simulink model "sensor_system"  (R2021b)
settings: Solver=VariableStepAuto  StartTime=0.0  StopTime=10  RelTol=1e-3
libraries: slpidlib x1, simulink x1
settings Model: Creator=mluser  LastModifiedBy=mluser

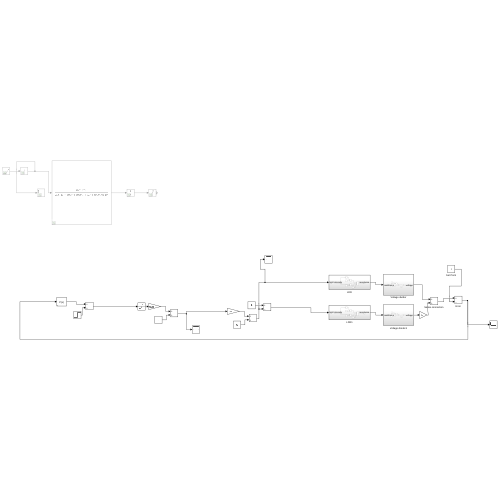
[thumbnail: Simulink's stored preview of the top-level diagram]
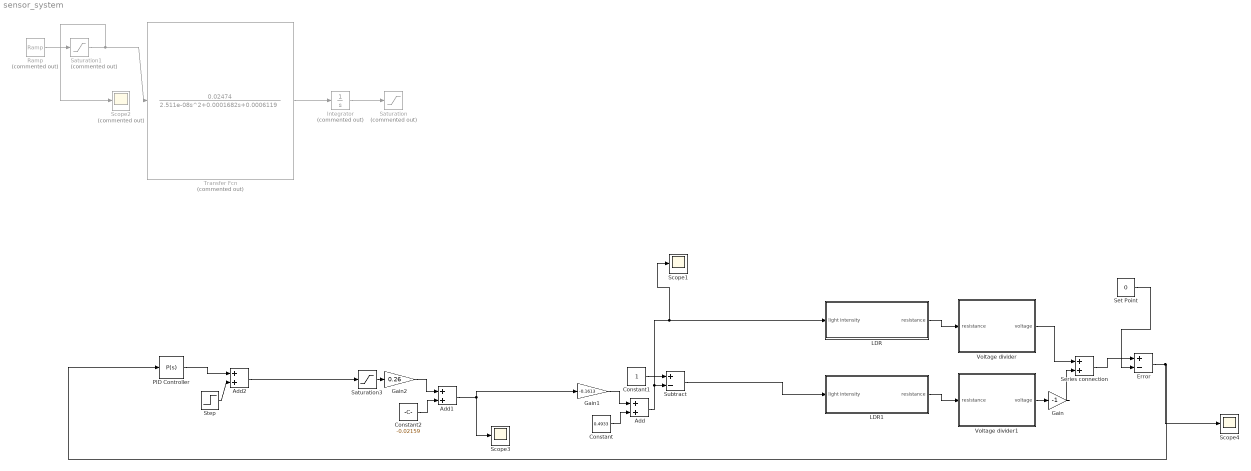
== system sensor_system ==
  Add : Sum
  Add1 : Sum
  Add2 : Sum
  Constant : Constant  Value=0.4933
  Constant1 : Constant
  Constant2 : Constant  Value=-0.02159
  Error : Sum  Inputs=+-
  Gain : Gain  Gain=-1
  Gain1 : Gain  Gain=-0.1613
  Gain2 : Gain  Gain=0.26
  Integrator : Integrator  Commented=on
  LDR : Subsystem
  LDR1 : Subsystem
  PID Controller : slpidlib/PID Controller  Controller=P  Form=Parallel  TimeDomain=Continuous-time  UseExternalTs=off  SampleTime=-1  IntegratorMethod=Forward Euler  FilterMethod=Forward Euler  ControllerParametersSource=internal  P=0.8  I=1  D=0.1  UseFilter=on  N=100  TunerSelectOption=Transfer Function Based (PID Tuner App)  InitialConditionSource=internal  InitialConditionForIntegrator=0  InitialConditionForFilter=0  DifferentiatorICPrevScaledInput=0  ExternalReset=none  TrackingMode=off  Kt=1  LimitOutput=off  SatLimitsSource=internal  UpperSaturationLimit=inf  LowerSaturationLimit=-inf  LinearizeAsGain=on  AntiWindupMode=none  Kb=1  POutMin=[]  POutMax=[]  IOutMin=[]  IOutMax=[]  DOutMin=[]  DOutMax=[]  NOutMin=[]  NOutMax=[]  SumOutMin=[]  SumOutMax=[]  SaturationOutMin=[]  SaturationOutMax=[]  PParamMin=[]  PParamMax=[]  IParamMin=[]  IParamMax=[]  DParamMin=[]  DParamMax=[]  NParamMin=[]  NParamMax=[]  KbParamMin=[]  KbParamMax=[]  KtParamMin=[]  KtParamMax=[]  KbOutMin=[]  KbOutMax=[]  KtOutMin=[]  KtOutMax=[]  IntegratorOutMin=[]  IntegratorOutMax=[]  FilterOutMin=[]  FilterOutMax=[]  SumI1OutMin=[]  SumI1OutMax=[]  SumI2OutMin=[]  SumI2OutMax=[]  SumI3OutMin=[]  SumI3OutMax=[]  SumI4OutMin=[]  SumI4OutMax=[]  SumDOutMin=[]  SumDOutMax=[]  DifferentiatorOutMin=[]  DifferentiatorOutMax=[]  FilterDiffOutCoefMin=[]  FilterDiffOutCoefMax=[]  ReciprocalOutMin=[]  ReciprocalOutMax=[]  SumDenOutMin=[]  SumDenOutMax=[]  SumNumOutMin=[]  SumNumOutMax=[]  DivideOutMin=[]  DivideOutMax=[]  UdiffTsProdOutMin=[]  UdiffTsProdOutMax=[]  NTsProdOutMin=[]  NTsProdOutMax=[]  UintegralTsProdOutMin=[]  UintegralTsProdOutMax=[]  UngainTsProdOutMin=[]  UngainTsProdOutMax=[]  IntegratorContinuousStateAttributes=''  IntegratorStateMustResolveToSignalObject=off  IntegratorRTWStateStorageClass=Auto  FilterContinuousStateAttributes=''  FilterStateMustResolveToSignalObject=off  FilterRTWStateStorageClass=Auto  ParallelPVariant=InternalParameters  IdealPVariant=Disabled  IVariant=Disabled  DVariant=Disabled  IntegratorVariant=Disabled  SatVariant=Disabled  AWVariant=Disabled  PCopyVariant=Disabled  TRVariant=Disabled  FdbkBlocksVariant=Forward  IdealPFdbkVariant=Disabled  SatFdbkVariant=Disabled  DerivativeFilterVariant=Disabled  NVariant=Disabled  NCopyVariant=Disabled_SignalSpec  FilterICVariant=Disabled  IntegratorICVariant=Disabled  ExternalResetVariant=Disabled  TRSumVariant=Passthrough  SumFdbkVariant=Disabled  SumVariant=Passthrough_P  TsampFilterVariant=InternalTs  TsampNgainVariant=Passthrough  TsampIntegralVariant=Disabled_SignalSpec  ExternalSaturationOutDataTypeStr=Inherit: Same as second input
  Ramp : simulink/Sources/Ramp  Commented=on  slope=2  start=0  InitialOutput=-12
  Saturation : Saturate  Commented=on  UpperLimit=pi  LowerLimit=-pi
  Saturation1 : Saturate  Commented=on  UpperLimit=12  LowerLimit=-12
  Saturation3 : Saturate  UpperLimit=12  LowerLimit=-12
  Scope1 : Scope
  Scope2 : Scope  Commented=on
  Scope3 : Scope
  Scope4 : Scope
  "Series connection " : Sum
  Set Point : Constant  Value=0
  Step : Step  Time=0.5  Before=-12  After=0  SampleTime=0
  Subtract : Sum  Inputs=+-
  Transfer Fcn : TransferFcn  Commented=on  Numerator=[0.02474]  Denominator=[2.511e-08 0.0001682 0.0006119]
  Voltage divider : Subsystem
  Voltage divider1 : Subsystem
  wires:
  LDR/1(resistance) -> Voltage divider/1(resistance)
  LDR1/1(resistance) -> Voltage divider1/1(resistance)
  Voltage divider/1(voltage) -> "Series connection "/1
  Voltage divider1/1(voltage) -> Gain/1
  Error/1 -> Scope4/1, PID Controller/1
  Gain/1 -> "Series connection "/2
  Transfer Fcn/1 -> Integrator/1
  Integrator/1 -> Saturation/1
  Constant/1 -> Add/2
  Gain1/1 -> Add/1
  Add/1 -> Scope1/1, LDR/1(light intensity), Subtract/2
  Subtract/1 -> LDR1/1(light intensity)
  Constant1/1 -> Subtract/1
  Ramp/1 -> Saturation1/1
  Saturation1/1 -> Scope2/1, Transfer Fcn/1
  Add1/1 -> Scope3/1, Gain1/1
  Constant2/1 -> Add1/2
  Gain2/1 -> Add1/1
  Saturation3/1 -> Gain2/1
  PID Controller/1 -> Add2/1
  Step/1 -> Add2/2
  Add2/1 -> Saturation3/1
  Set Point/1 -> Error/2
  "Series connection "/1 -> Error/1

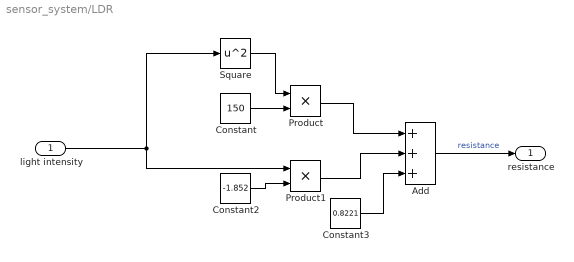
== system sensor_system/LDR ==
  light intensity : Inport
  Add : Sum  Inputs=+++
  Constant : Constant  Value=150
  Constant2 : Constant  Value=-1.852
  Constant3 : Constant  Value=0.8221
  Product : Product
  Product1 : Product
  Square : Math  Operator=square  SaturateOnIntegerOverflow=on
  resistance : Outport
  wires:
  Product/1 -> Add/1
  Constant2/1 -> Product1/2
  Add/1 -> resistance/1  "resistance"
  Square/1 -> Product/1
  Product1/1 -> Add/2
  light intensity/1 -> Square/1, Product1/1
  Constant/1 -> Product/2
  Constant3/1 -> Add/3

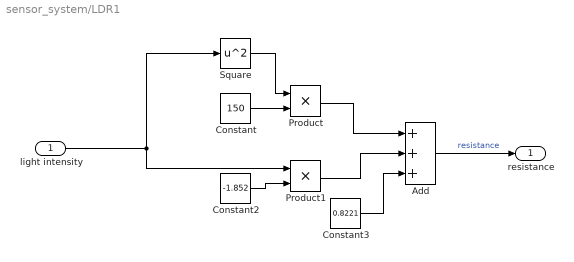
== system sensor_system/LDR1 ==
  light intensity : Inport
  Add : Sum  Inputs=+++
  Constant : Constant  Value=150
  Constant2 : Constant  Value=-1.852
  Constant3 : Constant  Value=0.8221
  Product : Product
  Product1 : Product
  Square : Math  Operator=square  SaturateOnIntegerOverflow=on
  resistance : Outport
  wires:
  Product/1 -> Add/1
  Constant2/1 -> Product1/2
  Add/1 -> resistance/1  "resistance"
  Square/1 -> Product/1
  Product1/1 -> Add/2
  light intensity/1 -> Square/1, Product1/1
  Constant/1 -> Product/2
  Constant3/1 -> Add/3

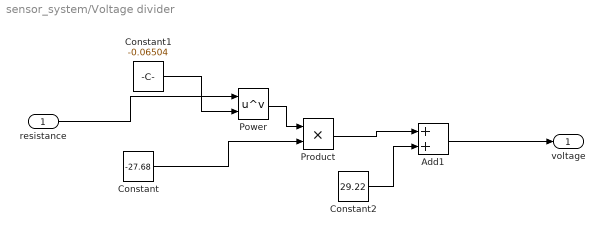
== system sensor_system/Voltage divider ==
  resistance : Inport
  Add1 : Sum
  Constant : Constant  Value=-27.68
  Constant1 : Constant  Value=-0.06504
  Constant2 : Constant  Value=29.22
  Power : Math  Operator=pow  SaturateOnIntegerOverflow=on
  Product : Product
  voltage : Outport
  wires:
  Power/1 -> Product/1
  Add1/1 -> voltage/1
  Product/1 -> Add1/1
  Constant2/1 -> Add1/2
  Constant/1 -> Product/2
  resistance/1 -> Power/1
  Constant1/1 -> Power/2

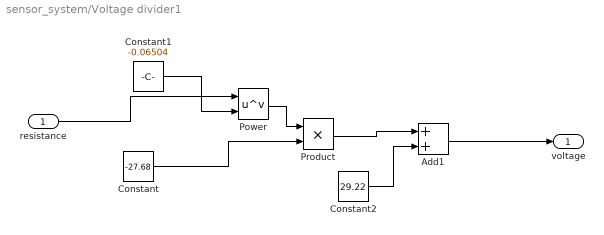
== system sensor_system/Voltage divider1 ==
  resistance : Inport
  Add1 : Sum
  Constant : Constant  Value=-27.68
  Constant1 : Constant  Value=-0.06504
  Constant2 : Constant  Value=29.22
  Power : Math  Operator=pow  SaturateOnIntegerOverflow=on
  Product : Product
  voltage : Outport
  wires:
  Power/1 -> Product/1
  Add1/1 -> voltage/1
  Product/1 -> Add1/1
  Constant2/1 -> Add1/2
  Constant/1 -> Product/2
  resistance/1 -> Power/1
  Constant1/1 -> Power/2
